simulink subsystem "BatteryHVDetailed_refsub_MultiModule"  (R2022a)
settings: Solver=VariableStepAuto  StartTime=0.0  StopTime=10.0  RelTol=1e-3
undefined symbols (not defined in the file or in its folder): batteryHV_multi_pack1, batteryHV_multi_pack2
libraries: fl_lib x139, nesl_utility x29, batteryModule_lib x12
(part 1 of 3)
settings Model: Creator=jjha  LastModifiedBy=isaacito
settings SolverCC: AlgebraicLoopSolver=TrustRegion
settings DebuggingCC: UnconnectedInputMsg=warning  UnconnectedOutputMsg=warning  UnconnectedLineMsg=warning
settings RTWCC: DLArmComputeVersion=19.05

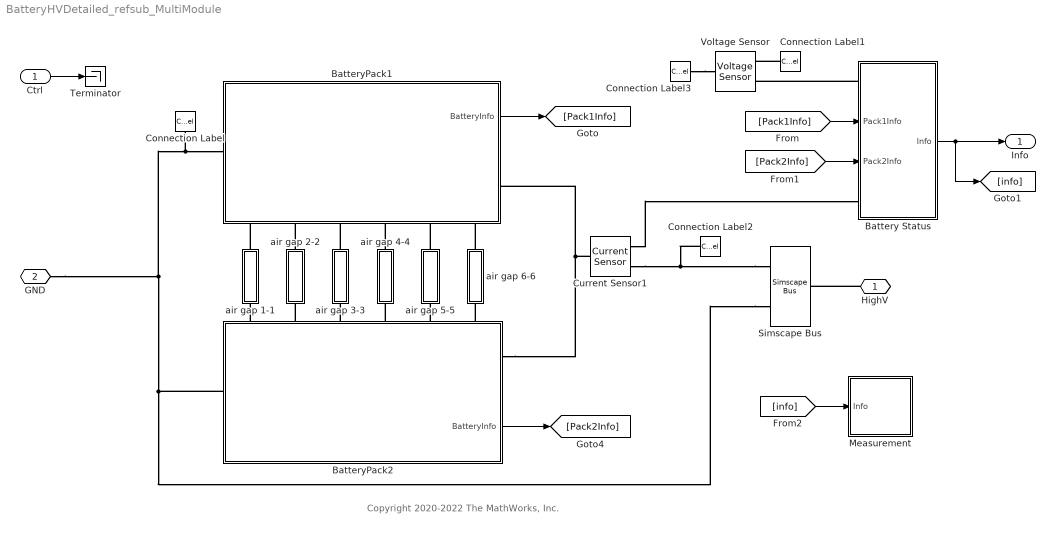
== system BatteryHVDetailed_refsub_MultiModule ==
  note: Copyright 2020-2022 The MathWorks, Inc.
  Ctrl : Inport
  Battery Status : Subsystem
      settings: PortSchema="{\"entries\":[{\"content\":{\"sides\":[{\"content\":{\"connectorIds\":[\"LConn1\",\"In1\",\"In2\",\"LConn2\"]},\"type\":\"ConnectorPlacement.EquallySpacedRectSide\",\"uuid\":\"ed01e2f8-b35f-4cf8-8a1f-a004924ddeb8\"},{\"content\":{\"connectorIds\":[\"Out1\"],\"side\":\"RIGHT\"},\"type\":\"ConnectorPlacement.EquallySpacedRectSide\",\"uuid\":\"7dc9989d-75e9-4ab2-9ee3-28d589c09f12\"},{\"content\":{\"connectorIds\":[],\"side\":\"TOP\"},\"type\":\"ConnectorPlacement.EquallySpacedRectSide\",\"uuid\":\"5d4fb4bf-c728-4f18-a915-de0993398bd4\"},{\"content\":{\"connectorIds\":[],\"side\":\"HIDDEN\"},\"type\":\"ConnectorPlacement.EquallySpacedRectSide\",\"uuid\":\"914bcd26-ac78-4b8d-9b0f-7ad78e1790ea\"}]},\"type\":\"ConnectorPlacement.EquallySpacedConnector\",\"uuid\":\"fc762cf8-918b-4a14-9282-253d1ee4be5d\"}],\"packageUris\":[\"http://schema.mathworks.com/mf0/Connector/R2020b\"],\"version\":\"1.0\"}"
  BatteryPack1 : Subsystem
      settings: PortSchema="{\"entries\":[{\"content\":{\"sides\":[{\"content\":{\"connectorIds\":[\"LConn1\"]},\"type\":\"ConnectorPlacement.EquallySpacedRectSide\",\"uuid\":\"b8d27d12-ba4e-497e-8eeb-93fb9beb614e\"},{\"content\":{\"connectorIds\":[\"Out1\",\"RConn1\"],\"side\":\"RIGHT\"},\"type\":\"ConnectorPlacement.EquallySpacedRectSide\",\"uuid\":\"3a767e09-1002-4db2-833d-9b3c14bcec7d\"},{\"content\":{\"connectorIds\":[],\"side\":\"TOP\"},\"type\":\"ConnectorPlacement.EquallySpacedRectSide\",\"uuid\":\"f8ad4e8a-2322-4ebd-b132-c16be085a9fd\"},{\"content\":{\"connectorIds\":[\"RConn2\",\"RConn3\",\"RConn4\",\"RConn5\",\"RConn6\",\"RConn7\"],\"side\":\"BOTTOM\"},\"type\":\"ConnectorPlacement.EquallySpacedRectSide\",\"uuid\":\"f73fd38f-dbed-4da5-b74f-fbadab7e811a\"},{\"content\":{\"connectorIds\":[],\"side\":\"HIDDEN\"},\"type\":\"ConnectorPlacement.EquallySpacedRectSide\",\"uuid\":\"26d95d03-e87b-489f-a99f-012a8d09d994\"}]},\"type\":\"ConnectorPlacement.EquallySpacedConnector\",\"uuid\":\"7600e896-e4bd-4da6-9432-0a1ab84cea55\"}],\"packageUris\":[\"http://schema.mathworks.com/mf0/Connector/R2020b\"],\"version\":\"1.0\"}"
      mask Display: image('Batterypack_SideView.png'); % Use "Edit Image" on toolstrip to change.
  BatteryPack2 : Subsystem
      settings: PortSchema="{\"entries\":[{\"content\":{\"sides\":[{\"content\":{\"connectorIds\":[\"LConn1\"]},\"type\":\"ConnectorPlacement.EquallySpacedRectSide\",\"uuid\":\"b8d27d12-ba4e-497e-8eeb-93fb9beb614e\"},{\"content\":{\"connectorIds\":[\"RConn1\",\"Out1\"],\"side\":\"RIGHT\"},\"type\":\"ConnectorPlacement.EquallySpacedRectSide\",\"uuid\":\"3a767e09-1002-4db2-833d-9b3c14bcec7d\"},{\"content\":{\"connectorIds\":[\"LConn2\",\"LConn3\",\"LConn4\",\"LConn5\",\"LConn6\",\"LConn7\"],\"side\":\"TOP\"},\"type\":\"ConnectorPlacement.EquallySpacedRectSide\",\"uuid\":\"f8ad4e8a-2322-4ebd-b132-c16be085a9fd\"},{\"content\":{\"connectorIds\":[],\"side\":\"BOTTOM\"},\"type\":\"ConnectorPlacement.EquallySpacedRectSide\",\"uuid\":\"f73fd38f-dbed-4da5-b74f-fbadab7e811a\"},{\"content\":{\"connectorIds\":[],\"side\":\"HIDDEN\"},\"type\":\"ConnectorPlacement.EquallySpacedRectSide\",\"uuid\":\"26d95d03-e87b-489f-a99f-012a8d09d994\"}]},\"type\":\"ConnectorPlacement.EquallySpacedConnector\",\"uuid\":\"7600e896-e4bd-4da6-9432-0a1ab84cea55\"}],\"packageUris\":[\"http://schema.mathworks.com/mf0/Connector/R2020b\"],\"version\":\"1.0\"}"
      mask Display: image('Batterypack_SideView.png'); % Use "Edit Image" on toolstrip to change.
  Connection Label : ConnectionLabel  Label=BatNeg
  Connection Label1 : ConnectionLabel  Label=BatNeg
  Connection Label2 : ConnectionLabel  Label=BatPos
  Connection Label3 : ConnectionLabel  Label=BatPos
  Current Sensor1 : fl_lib/Electrical/Electrical Sensors/Current Sensor
      settings: SourceProductBaseCode=PW,SS,VE
  Measurement : Subsystem
  Simscape Bus : SimscapeBus  HierarchyStrings=plus;minus
  Terminator : Terminator
  Voltage Sensor : fl_lib/Electrical/Electrical Sensors/Voltage Sensor
      settings: SourceProductBaseCode=PW,SS,VE
  air gap 1-1 : Subsystem
  air gap 2-2 : Subsystem
  air gap 3-3 : Subsystem
  air gap 4-4 : Subsystem
  air gap 5-5 : Subsystem
  air gap 6-6 : Subsystem
  HighV : PMIOPort  Side=Right
  GND : PMIOPort  Port=2  Side=Left
  Info : Outport
  wires:
  Battery Status/1(Info) -> Info/1, [info]
  BatteryPack2/1(BatteryInfo) -> [Pack2Info]
  Ctrl/1 -> Terminator/1
  BatteryPack1/1(BatteryInfo) -> [Pack1Info]
  [Pack1Info] -> Battery Status/1(Pack1Info)
  [Pack2Info] -> Battery Status/2(Pack2Info)
  [info] -> Measurement/1(Info)
  connections:
  BatteryPack2/RConn1 -- Current Sensor1/LConn1 -- BatteryPack1/RConn1
  Simscape Bus/LConn2 -- Connection Label/LConn1 -- BatteryPack1/LConn1 -- GND/RConn1 -- BatteryPack2/LConn1
  Simscape Bus/LConn1 -- Connection Label2/LConn1 -- Current Sensor1/RConn2
  HighV/RConn1 -- Simscape Bus/RConn1
  BatteryPack2/LConn7 -- air gap 6-6/RConn1
  Battery Status/LConn1 -- Voltage Sensor/RConn1
  Current Sensor1/RConn1 -- Battery Status/LConn2
  BatteryPack2/LConn2 -- air gap 1-1/RConn1
  BatteryPack2/LConn3 -- air gap 2-2/RConn1
  BatteryPack2/LConn4 -- air gap 3-3/RConn1
  BatteryPack2/LConn5 -- air gap 4-4/RConn1
  BatteryPack2/LConn6 -- air gap 5-5/RConn1
  air gap 5-5/LConn1 -- BatteryPack1/RConn6
  air gap 4-4/LConn1 -- BatteryPack1/RConn5
  air gap 6-6/LConn1 -- BatteryPack1/RConn7
  air gap 2-2/LConn1 -- BatteryPack1/RConn3
  air gap 1-1/LConn1 -- BatteryPack1/RConn2
  air gap 3-3/LConn1 -- BatteryPack1/RConn4
  Connection Label1/LConn1 -- Voltage Sensor/RConn2
  Connection Label3/LConn1 -- Voltage Sensor/LConn1

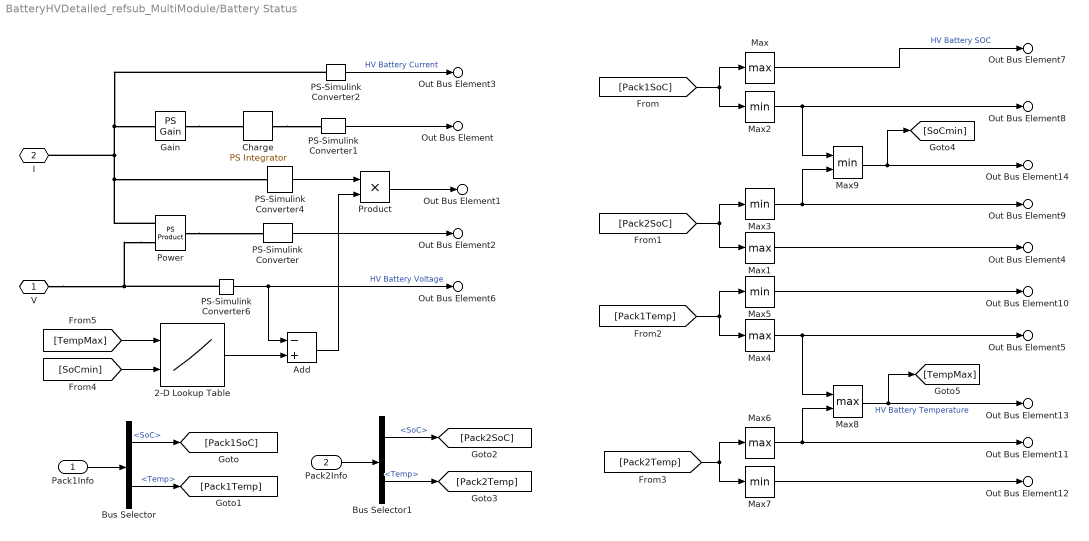
== system BatteryHVDetailed_refsub_MultiModule/Battery Status ==
  Pack1Info : Inport
  Pack2Info : Inport  Port=2
  2-D Lookup Table : Lookup_n-D  BreakpointsForDimension1=batteryHV_multi_pack1.batterySOC_LUT  BreakpointsForDimension2=batteryHV_multi_pack1.batteryTemp_LUT  Table=batteryHV_multi_pack1.batteryEm_LUT  InternalRulePriority=Speed  RndMeth=Simplest
      settings: InputPortMap=u0,u1
  Add : Sum  Inputs=-+
  Bus Selector : BusSelector  OutputSignals=SoC,Temp
  Bus Selector1 : BusSelector  OutputSignals=SoC,Temp
  Charge : fl_lib/Physical Signals/Linear Operators/PS Integrator  reset_method=foundation.enum.IntegratorResetSpec.None  initial_condition_spec=foundation.enum.IntegratorICSpec.Internal  x0=batteryHV_multi_other.batteryPackAhr_ini A*hr
      settings: SourceProductBaseCode=PW,SS,VE
  Gain : fl_lib/Physical Signals/Functions/PS Gain  gain=-1
      settings: AttributesFormatString=%<gain>  SourceProductBaseCode=PW,SS,VE
  Max{,1,4,6} (4 alike) : MinMax  Function=max  ZeroCross=off
  Max{2..3,5,7} (4 alike) : MinMax  ZeroCross=off
  Max8 : MinMax  Function=max  Inputs=2
  Max9 : MinMax  Inputs=2
  PS-Simulink Converter : nesl_utility/PS-Simulink Converter  PhysicalDomain=network_engine_domain  SubClassName=ps_output  LeftPortType=input  RightPortType=output  PseudoPeriodic=off  Frequencies=[]  VectorFormat=1-D array  Unit=kW  AffineConversion=off
      settings: SourceProductBaseCode=SS,PW,VE
  PS-Simulink Converter1 : nesl_utility/PS-Simulink Converter  PhysicalDomain=network_engine_domain  SubClassName=ps_output  LeftPortType=input  RightPortType=output  PseudoPeriodic=off  Frequencies=[]  VectorFormat=1-D array  Unit=A*hr  AffineConversion=off
      settings: SourceProductBaseCode=SS,PW,VE
  PS-Simulink Converter2 : nesl_utility/PS-Simulink Converter  PhysicalDomain=network_engine_domain  SubClassName=ps_output  LeftPortType=input  RightPortType=output  PseudoPeriodic=off  Frequencies=[]  VectorFormat=1-D array  Unit=A  AffineConversion=off
      settings: SourceProductBaseCode=SS,PW,VE
  PS-Simulink Converter4 : nesl_utility/PS-Simulink Converter  PhysicalDomain=network_engine_domain  SubClassName=ps_output  LeftPortType=input  RightPortType=output  PseudoPeriodic=off  Frequencies=[]  VectorFormat=1-D array  Unit=A  AffineConversion=off
      settings: SourceProductBaseCode=SS,PW,VE
  PS-Simulink Converter6 : nesl_utility/PS-Simulink Converter  PhysicalDomain=network_engine_domain  SubClassName=ps_output  LeftPortType=input  RightPortType=output  PseudoPeriodic=off  Frequencies=[]  VectorFormat=1-D array  Unit=V  AffineConversion=off
      settings: SourceProductBaseCode=SS,PW,VE
  Power : fl_lib/Physical Signals/Functions/PS Product
      settings: SourceProductBaseCode=PW,SS,VE
  Product : Product
  V : PMIOPort  Side=Left
  I : PMIOPort  Port=2  Side=Left
  Out Bus Element : Outport  PortName=Info  Element=Charge
      settings: AttributesFormatString=%<Unit>
  Out Bus Element1 : Outport  PortName=Info  Element=PowerLoss
      settings: AttributesFormatString=%<Unit>
  Out Bus Element2 : Outport  PortName=Info  Element=Power
      settings: AttributesFormatString=%<Unit>
  Out Bus Element3 : Outport  PortName=Info  Element=Current
      settings: AttributesFormatString=%<Unit>
  Out Bus Element4 : Outport  PortName=Info  Element=SoC2Max
      settings: AttributesFormatString=%<Unit>
  Out Bus Element5 : Outport  PortName=Info  Element=Temp1Max
      settings: AttributesFormatString=%<Unit>
  Out Bus Element6 : Outport  PortName=Info  Element=Voltage
      settings: AttributesFormatString=%<Unit>
  Out Bus Element7 : Outport  PortName=Info  Element=SoC1Max
      settings: AttributesFormatString=%<Unit>
  Out Bus Element8 : Outport  PortName=Info  Element=SoC1Min
      settings: AttributesFormatString=%<Unit>
  Out Bus Element9 : Outport  PortName=Info  Element=SoC2Min
      settings: AttributesFormatString=%<Unit>
  Out Bus Element10 : Outport  PortName=Info  Element=Temp1Min
      settings: AttributesFormatString=%<Unit>
  Out Bus Element11 : Outport  PortName=Info  Element=Temp2Max
      settings: AttributesFormatString=%<Unit>
  Out Bus Element12 : Outport  PortName=Info  Element=Temp2Min
      settings: AttributesFormatString=%<Unit>
  Out Bus Element13 : Outport  PortName=Info  Element=Temp
      settings: AttributesFormatString=%<Unit>
  Out Bus Element14 : Outport  PortName=Info  Element=SOC
      settings: AttributesFormatString=%<Unit>
  wires:
  Max8/1 -> Out Bus Element13/1, [TempMax]  "HV Battery Temperature"
  Max9/1 -> Out Bus Element14/1, [SoCmin]
  Add/1 -> Product/2
  PS-Simulink Converter4/1 -> Product/1
  2-D Lookup Table/1 -> Add/2
  [TempMax] -> 2-D Lookup Table/1
  [SoCmin] -> 2-D Lookup Table/2
  Max3/1 -> Out Bus Element9/1, Max9/2
  Max6/1 -> Out Bus Element11/1, Max8/2
  Bus Selector1/2 -> [Pack2Temp]  "<Temp>"
  Bus Selector1/1 -> [Pack2SoC]  "<SoC>"
  Bus Selector/2 -> [Pack1Temp]  "<Temp>"
  Bus Selector/1 -> [Pack1SoC]  "<SoC>"
  Pack2Info/1 -> Bus Selector1/1
  Pack1Info/1 -> Bus Selector/1
  PS-Simulink Converter6/1 -> Out Bus Element6/1, Add/1  "HV Battery Voltage"
  PS-Simulink Converter2/1 -> Out Bus Element3/1  "HV Battery Current"
  PS-Simulink Converter/1 -> Out Bus Element2/1
  PS-Simulink Converter1/1 -> Out Bus Element/1
  Product/1 -> Out Bus Element1/1
  [Pack1SoC] -> Max2/1, Max/1
  [Pack2SoC] -> Max1/1, Max3/1
  [Pack1Temp] -> Max4/1, Max5/1
  [Pack2Temp] -> Max7/1, Max6/1
  Max1/1 -> Out Bus Element4/1
  Max/1 -> Out Bus Element7/1  "HV Battery SOC"
  Max2/1 -> Out Bus Element8/1, Max9/1
  Max4/1 -> Out Bus Element5/1, Max8/1
  Max5/1 -> Out Bus Element10/1
  Max7/1 -> Out Bus Element12/1
  connections:
  Gain/RConn1 -- Charge/LConn1
  Charge/RConn1 -- PS-Simulink Converter1/LConn1
  Power/RConn1 -- PS-Simulink Converter/LConn1
  Power/LConn1 -- PS-Simulink Converter6/LConn1 -- V/RConn1
  I/RConn1 -- PS-Simulink Converter4/LConn1 -- Power/LConn2 -- Gain/LConn1 -- PS-Simulink Converter2/LConn1

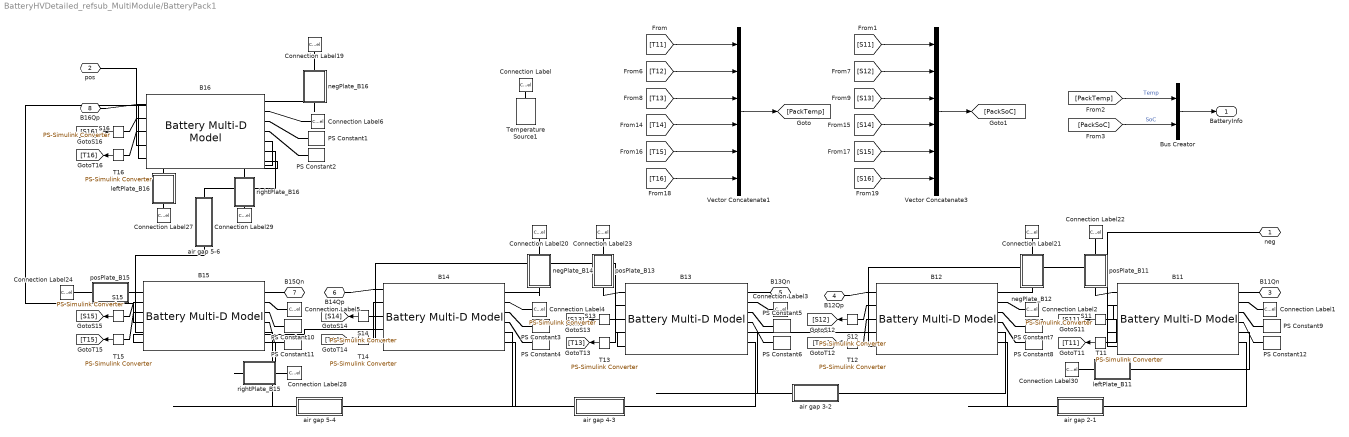
== system BatteryHVDetailed_refsub_MultiModule/BatteryPack1 ==
  B{11..14} (4 alike) : batteryModule_lib/Battery Multi-D Model  modelComplexity=batteryModule.batteryAbstractionLevel.grouped  LUTpointsTemp=batteryHV_multi_pack1.batteryTemp_LUT K  cellAH=batteryHV_multi_pack1.batteryCharge_Ahr A*hr  LUTpointsSOC=batteryHV_multi_pack1.batterySOC_LUT  V0_mat=batteryHV_multi_pack1.batteryEm_LUT V  prm_dir=ee.enum.battery.prm_dir.noCurrentDirectionality  R0_mat=batteryHV_multi_pack1.batteryR0_LUT Ohm  R0_dis_mat=[.03, .015, .002; .04, .017, .008; .039, .012, .006; .027, .013, .021] Ohm  R0_ch_mat=[.03, .015, .002; .04, .017, .008; .039, .012, .006; .027, .013, .021] Ohm  prm_leak=ee.enum.battery.prm_leak.disabled  Rleak_vec=[8000, 7000, 6000] Ohm  extrapolation_option=simscape.enum.extrapolation.nearest  prm_dyn=ee.enum.battery.prm_dyn.rc1  R1_mat=batteryHV_multi_pack1.batteryR1_LUT Ohm  tau1_mat=batteryHV_multi_pack1.batteryTau1_LUT s  R2_mat=[.014, .382, .407; .028, .006, .007; .014, .007, .006; .333, .956, .912] Ohm  tau2_mat=[1, 44, 5644; 11, 24, 506; 2, 14, 330; 3310, 13419, 30216] s  R3_mat=[.014, .382, .407; .028, .006, .007; .014, .007, .006; .333, .956, .912] Ohm  tau3_mat=[1, 44, 5644; 11, 24, 506; 2, 14, 330; 3310, 13419, 30216] s  R4_mat=[.014, .382, .407; .028, .006, .007; .014, .007, .006; .333, .956, .912] Ohm  tau4_mat=[1, 44, 5644; 11, 24, 506; 2, 14, 330; 3310, 13419, 30216] s  R5_mat=[.014, .382, .407; .028, .006, .007; .014, .007, .006; .333, .956, .912] Ohm  tau5_mat=[1, 44, 5644; 11, 24, 506; 2, 14, 330; 3310, 13419, 30216] s  prm_fade=ee.enum.battery.prm_fade.equations  N0=100  dV0=0  dR0=0  dAH=0  dRleak=0  dR1=0  dR2=0  dR3=0  dR4=0  dR5=0  N0vec=[100, 200, 300]  Tfadevec=[298.15, 323.15] K  dV0vec=[0, 0, 0]  dR0vec=[0, 0, 0]  dAHvec=[0, 0, 0]  dRleakvec=[0, 0, 0]  dR1vec=[0, 0, 0]  dR2vec=[0, 0, 0]  dR3vec=[0, 0, 0]  dR4vec=[0, 0, 0]  dR5vec=[0, 0, 0]  dV0mat=[0, 0; 0, 0; 0, 0]  dR0mat=[0, 0; 0, 0; 0, 0]  dAHmat=[0, 0; 0, 0; 0, 0]  dRleakmat=[0, 0; 0, 0; 0, 0]  dR1mat=[0, 0; 0, 0; 0, 0]  dR2mat=[0, 0; 0, 0; 0, 0]  dR3mat=[0, 0; 0, 0; 0, 0]  dR4mat=[0, 0; 0, 0; 0, 0]  dR5mat=[0, 0; 0, 0; 0, 0]  cellThermalMass=batteryHV_multi_pack1.batteryCell_mass*batteryHV_multi_pack1.batteryCell_cp J/K  cellThermalCond=batteryHV_multi_pack1.batteryThermal_K1 W/(m*K)  cellThermalCond_inPlane=batteryHV_multi_pack1.batteryThermal_K2 W/(m*K)  Ns=batteryHV_multi_pack1.batteryNs  Np=batteryHV_multi_pack1.batteryNp  cellTypeSelection=batteryModule.batteryTypeSelection.pouch  cellHeight=batteryHV_multi_pack1.batteryCell_H m  cellWidth=batteryHV_multi_pack1.batteryCell_W m  cellThickness=batteryHV_multi_pack1.batteryCell_T m  cellDiameter=0.018 m  cellCylinLine=3  moduleExternalR=batteryHV_multi_pack1.battery_extR Ohm  moduleCellBalancing=batteryModule.batteryCellBalancing.none  passiveShuntR=50 Ohm  passiveSWclosedR=0.01 Ohm  passiveSWopenCond=1e-8 1/Ohm  passiveSWthreshold=0.5  moduleCellVoltages=batteryModule.batteryCellVoltages.no  thermalManagement=batteryModule.batteryCoolingSystem.thermalPort  cellHeatTrCoeff=1 W/(m^2 * K)  thermal_moduleBottom=batteryModule.batteryThermalPortSelection.thermalLUT  htc_bottom=1 W/(m^2 * K)  moduleCooling_b=batteryHV_multi_pack1.batteryModuleBottomHTC W/K  LUTpointsFlowrate_b=batteryHV_multi_pack1.batteryCoolant_flow kg/s  LUTpointsTemp_b=batteryHV_multi_pack1.batteryTemp_LUT K  thermal_moduleTop=batteryModule.batteryThermalPortSelection.convectionBC  htc_top=batteryHV_multi_pack1.batteryModuleTopHTC W/(m^2 * K)  moduleCooling_t=batteryHV_multi_pack1.batteryCoolantHTC W/K  LUTpointsFlowrate_t=batteryHV_multi_pack1.batteryCoolant_flow kg/s  LUTpointsTemp_t=batteryHV_multi_pack1.batteryTemp_LUT K  thermal_moduleRight=batteryModule.batteryThermalPortSelection.thermalPortLumped  htc_right=1 W/(m^2 * K)  moduleCooling_r=zeros(3,6,batteryHV_multi_pack1.batteryNs*batteryHV_multi_pack1.batteryNp) W/K  LUTpointsFlowrate_r=[.01, .02, .03, .04, .05, .06] kg/s  LUTpointsTemp_r=[273.15, 298.15, 323.15] K  thermal_moduleLeft=batteryModule.batteryThermalPortSelection.thermalPortLumped  htc_left=1 W/(m^2 * K)  moduleCooling_l=zeros(3,6,batteryHV_multi_pack1.batteryNs*batteryHV_multi_pack1.batteryNp) W/K  LUTpointsFlowrate_l=[.01, .02, .03, .04, .05, .06] kg/s  LUTpointsTemp_l=[273.15, 298.15, 323.15] K  thermal_modulePos=batteryModule.batteryThermalPortSelection.thermalPortLumped  htc_pos=1 W/(m^2 * K)  moduleCooling_p=zeros(3,6,batteryHV_multi_pack1.batteryNs*batteryHV_multi_pack1.batteryNp) W/K  LUTpointsFlowrate_p=[.01, .02, .03, .04, .05, .06] kg/s  LUTpointsTemp_p=[273.15, 298.15, 323.15] K  thermal_moduleNeg=batteryModule.batteryThermalPortSelection.thermalPortLumped  htc_neg=1 W/(m^2 * K)  moduleCooling_n=zeros(3,6,batteryHV_multi_pack1.batteryNs*batteryHV_multi_pack1.batteryNp) W/K  LUTpointsFlowrate_n=[.01, .02, .03, .04, .05, .06] kg/s  LUTpointsTemp_n=[273.15, 298.15, 323.15] K  moduleExtHeat=batteryHV_multi_pack1.batteryModuleExtHeat W  cellTemp=batteryHV_multi_pack1.batteryModuleCellT_ini K  cellSOC=batteryHV_multi_pack1.batteryModuleCellSOC_ini  moduleCellAHpercentVar=batteryHV_multi_pack1.batteryModuleCellAhr_ini  moduleCellLeakPercentVar=ones(1, 10)  moduleCellR0PercentVar=batteryHV_multi_pack1.batteryModuleCellR0_ini
      settings: InternalSimscapePortConfiguration="{\"Bottom\":[{\"id\":\"Ql\",\"label\":\"Ql\",\"type\":\"foundation.thermal.thermal\"},{\"id\":\"Qr\",\"label\":\"Qr\",\"type\":\"foundation.thermal.thermal\"}],\"Left\":[{\"id\":\"Qp\",\"label\":\"Qp\",\"type\":\"foundation.thermal.thermal\"},{\"id\":\"outputCellSOC\",\"label\":\"SOC\",\"type\":\"output\"},{\"id\":\"outputCellTemp\",\"label\":\"Temp\",\"type\":\"output\"}],\"Right\":[{\"id\":\"Qn\",\"label\":\"Qn\",\"type\":\"foundation.thermal.thermal\"},{\"id\":\"H\",\"label\":\"Amb\",\"type\":\"foundation.thermal.thermal\"},{\"id\":\"frac_b\",\"label\":\"FlwR\",\"type\":\"input\"},{\"id\":\"delT_b\",\"label\":\"FlwT\",\"type\":\"input\"}],\"Top\":[{\"id\":\"p\",\"label\":\"pos\",\"type\":\"foundation.electrical.electrical\"},{\"id\":\"n\",\"label\":\"neg\",\"type\":\"foundation.electrical.electrical\"}]}"
  B15 : batteryModule_lib/Battery Multi-D Model  modelComplexity=batteryModule.batteryAbstractionLevel.grouped  LUTpointsTemp=batteryHV_multi_pack1.batteryTemp_LUT K  cellAH=batteryHV_multi_pack1.batteryCharge_Ahr A*hr  LUTpointsSOC=batteryHV_multi_pack1.batterySOC_LUT  V0_mat=batteryHV_multi_pack1.batteryEm_LUT V  prm_dir=ee.enum.battery.prm_dir.noCurrentDirectionality  R0_mat=batteryHV_multi_pack1.batteryR0_LUT Ohm  R0_dis_mat=[.03, .015, .002; .04, .017, .008; .039, .012, .006; .027, .013, .021] Ohm  R0_ch_mat=[.03, .015, .002; .04, .017, .008; .039, .012, .006; .027, .013, .021] Ohm  prm_leak=ee.enum.battery.prm_leak.disabled  Rleak_vec=[8000, 7000, 6000] Ohm  extrapolation_option=simscape.enum.extrapolation.nearest  prm_dyn=ee.enum.battery.prm_dyn.rc1  R1_mat=batteryHV_multi_pack1.batteryR1_LUT Ohm  tau1_mat=batteryHV_multi_pack1.batteryTau1_LUT s  R2_mat=[.014, .382, .407; .028, .006, .007; .014, .007, .006; .333, .956, .912] Ohm  tau2_mat=[1, 44, 5644; 11, 24, 506; 2, 14, 330; 3310, 13419, 30216] s  R3_mat=[.014, .382, .407; .028, .006, .007; .014, .007, .006; .333, .956, .912] Ohm  tau3_mat=[1, 44, 5644; 11, 24, 506; 2, 14, 330; 3310, 13419, 30216] s  R4_mat=[.014, .382, .407; .028, .006, .007; .014, .007, .006; .333, .956, .912] Ohm  tau4_mat=[1, 44, 5644; 11, 24, 506; 2, 14, 330; 3310, 13419, 30216] s  R5_mat=[.014, .382, .407; .028, .006, .007; .014, .007, .006; .333, .956, .912] Ohm  tau5_mat=[1, 44, 5644; 11, 24, 506; 2, 14, 330; 3310, 13419, 30216] s  prm_fade=ee.enum.battery.prm_fade.equations  N0=100  dV0=0  dR0=0  dAH=0  dRleak=0  dR1=0  dR2=0  dR3=0  dR4=0  dR5=0  N0vec=[100, 200, 300]  Tfadevec=[298.15, 323.15] K  dV0vec=[0, 0, 0]  dR0vec=[0, 0, 0]  dAHvec=[0, 0, 0]  dRleakvec=[0, 0, 0]  dR1vec=[0, 0, 0]  dR2vec=[0, 0, 0]  dR3vec=[0, 0, 0]  dR4vec=[0, 0, 0]  dR5vec=[0, 0, 0]  dV0mat=[0, 0; 0, 0; 0, 0]  dR0mat=[0, 0; 0, 0; 0, 0]  dAHmat=[0, 0; 0, 0; 0, 0]  dRleakmat=[0, 0; 0, 0; 0, 0]  dR1mat=[0, 0; 0, 0; 0, 0]  dR2mat=[0, 0; 0, 0; 0, 0]  dR3mat=[0, 0; 0, 0; 0, 0]  dR4mat=[0, 0; 0, 0; 0, 0]  dR5mat=[0, 0; 0, 0; 0, 0]  cellThermalMass=batteryHV_multi_pack1.batteryCell_mass*batteryHV_multi_pack1.batteryCell_cp J/K  cellThermalCond=batteryHV_multi_pack1.batteryThermal_K1 W/(m*K)  cellThermalCond_inPlane=batteryHV_multi_pack1.batteryThermal_K2 W/(m*K)  Ns=batteryHV_multi_pack1.batteryNs  Np=batteryHV_multi_pack1.batteryNp  cellTypeSelection=batteryModule.batteryTypeSelection.pouch  cellHeight=batteryHV_multi_pack1.batteryCell_H m  cellWidth=batteryHV_multi_pack1.batteryCell_W m  cellThickness=batteryHV_multi_pack1.batteryCell_T m  cellDiameter=0.018 m  cellCylinLine=3  moduleExternalR=batteryHV_multi_pack1.battery_extR Ohm  moduleCellBalancing=batteryModule.batteryCellBalancing.none  passiveShuntR=50 Ohm  passiveSWclosedR=0.01 Ohm  passiveSWopenCond=1e-8 1/Ohm  passiveSWthreshold=0.5  moduleCellVoltages=batteryModule.batteryCellVoltages.no  thermalManagement=batteryModule.batteryCoolingSystem.thermalPort  cellHeatTrCoeff=1 W/(m^2 * K)  thermal_moduleBottom=batteryModule.batteryThermalPortSelection.thermalLUT  htc_bottom=1 W/(m^2 * K)  moduleCooling_b=batteryHV_multi_pack1.batteryModuleBottomHTC W/K  LUTpointsFlowrate_b=batteryHV_multi_pack1.batteryCoolant_flow kg/s  LUTpointsTemp_b=batteryHV_multi_pack1.batteryTemp_LUT K  thermal_moduleTop=batteryModule.batteryThermalPortSelection.thermalPortLumped  htc_top=batteryHV_multi_pack1.batteryModuleTopHTC W/(m^2 * K)  moduleCooling_t=batteryHV_multi_pack1.batteryCoolantHTC W/K  LUTpointsFlowrate_t=batteryHV_multi_pack1.batteryCoolant_flow kg/s  LUTpointsTemp_t=batteryHV_multi_pack1.batteryTemp_LUT K  thermal_moduleRight=batteryModule.batteryThermalPortSelection.thermalPortLumped  htc_right=1 W/(m^2 * K)  moduleCooling_r=zeros(3,6,batteryHV_multi_pack1.batteryNs*batteryHV_multi_pack1.batteryNp) W/K  LUTpointsFlowrate_r=[.01, .02, .03, .04, .05, .06] kg/s  LUTpointsTemp_r=[273.15, 298.15, 323.15] K  thermal_moduleLeft=batteryModule.batteryThermalPortSelection.thermalPortLumped  htc_left=1 W/(m^2 * K)  moduleCooling_l=zeros(3,6,batteryHV_multi_pack1.batteryNs*batteryHV_multi_pack1.batteryNp) W/K  LUTpointsFlowrate_l=[.01, .02, .03, .04, .05, .06] kg/s  LUTpointsTemp_l=[273.15, 298.15, 323.15] K  thermal_modulePos=batteryModule.batteryThermalPortSelection.thermalPortLumped  htc_pos=1 W/(m^2 * K)  moduleCooling_p=zeros(3,6,batteryHV_multi_pack1.batteryNs*batteryHV_multi_pack1.batteryNp) W/K  LUTpointsFlowrate_p=[.01, .02, .03, .04, .05, .06] kg/s  LUTpointsTemp_p=[273.15, 298.15, 323.15] K  thermal_moduleNeg=batteryModule.batteryThermalPortSelection.thermalPortLumped  htc_neg=1 W/(m^2 * K)  moduleCooling_n=zeros(3,6,batteryHV_multi_pack1.batteryNs*batteryHV_multi_pack1.batteryNp) W/K  LUTpointsFlowrate_n=[.01, .02, .03, .04, .05, .06] kg/s  LUTpointsTemp_n=[273.15, 298.15, 323.15] K  moduleExtHeat=batteryHV_multi_pack1.batteryModuleExtHeat W  cellTemp=batteryHV_multi_pack1.batteryModuleCellT_ini K  cellSOC=batteryHV_multi_pack1.batteryModuleCellSOC_ini  moduleCellAHpercentVar=batteryHV_multi_pack1.batteryModuleCellAhr_ini  moduleCellLeakPercentVar=ones(1, 10)  moduleCellR0PercentVar=batteryHV_multi_pack1.batteryModuleCellR0_ini
      settings: InternalSimscapePortConfiguration="{\"Bottom\":[{\"id\":\"Ql\",\"label\":\"Ql\",\"type\":\"foundation.thermal.thermal\"},{\"id\":\"Qr\",\"label\":\"Qr\",\"type\":\"foundation.thermal.thermal\"}],\"Left\":[{\"id\":\"Qp\",\"label\":\"Qp\",\"type\":\"foundation.thermal.thermal\"},{\"id\":\"outputCellSOC\",\"label\":\"SOC\",\"type\":\"output\"},{\"id\":\"outputCellTemp\",\"label\":\"Temp\",\"type\":\"output\"}],\"Right\":[{\"id\":\"Qn\",\"label\":\"Qn\",\"type\":\"foundation.thermal.thermal\"},{\"id\":\"H\",\"label\":\"Amb\",\"type\":\"foundation.thermal.thermal\"},{\"id\":\"frac_b\",\"label\":\"FlwR\",\"type\":\"input\"},{\"id\":\"delT_b\",\"label\":\"FlwT\",\"type\":\"input\"}],\"Top\":[{\"id\":\"p\",\"label\":\"pos\",\"type\":\"foundation.electrical.electrical\"},{\"id\":\"Qt\",\"label\":\"Qt\",\"type\":\"foundation.thermal.thermal\"},{\"id\":\"n\",\"label\":\"neg\",\"type\":\"foundation.electrical.electrical\"}]}"
  B16 : batteryModule_lib/Battery Multi-D Model  modelComplexity=batteryModule.batteryAbstractionLevel.grouped  LUTpointsTemp=batteryHV_multi_pack1.batteryTemp_LUT K  cellAH=batteryHV_multi_pack1.batteryCharge_Ahr A*hr  LUTpointsSOC=batteryHV_multi_pack1.batterySOC_LUT  V0_mat=batteryHV_multi_pack1.batteryEm_LUT V  prm_dir=ee.enum.battery.prm_dir.noCurrentDirectionality  R0_mat=batteryHV_multi_pack1.batteryR0_LUT Ohm  R0_dis_mat=[.03, .015, .002; .04, .017, .008; .039, .012, .006; .027, .013, .021] Ohm  R0_ch_mat=[.03, .015, .002; .04, .017, .008; .039, .012, .006; .027, .013, .021] Ohm  prm_leak=ee.enum.battery.prm_leak.disabled  Rleak_vec=[8000, 7000, 6000] Ohm  extrapolation_option=simscape.enum.extrapolation.nearest  prm_dyn=ee.enum.battery.prm_dyn.rc1  R1_mat=batteryHV_multi_pack1.batteryR1_LUT Ohm  tau1_mat=batteryHV_multi_pack1.batteryTau1_LUT s  R2_mat=[.014, .382, .407; .028, .006, .007; .014, .007, .006; .333, .956, .912] Ohm  tau2_mat=[1, 44, 5644; 11, 24, 506; 2, 14, 330; 3310, 13419, 30216] s  R3_mat=[.014, .382, .407; .028, .006, .007; .014, .007, .006; .333, .956, .912] Ohm  tau3_mat=[1, 44, 5644; 11, 24, 506; 2, 14, 330; 3310, 13419, 30216] s  R4_mat=[.014, .382, .407; .028, .006, .007; .014, .007, .006; .333, .956, .912] Ohm  tau4_mat=[1, 44, 5644; 11, 24, 506; 2, 14, 330; 3310, 13419, 30216] s  R5_mat=[.014, .382, .407; .028, .006, .007; .014, .007, .006; .333, .956, .912] Ohm  tau5_mat=[1, 44, 5644; 11, 24, 506; 2, 14, 330; 3310, 13419, 30216] s  prm_fade=ee.enum.battery.prm_fade.equations  N0=100  dV0=0  dR0=0  dAH=0  dRleak=0  dR1=0  dR2=0  dR3=0  dR4=0  dR5=0  N0vec=[100, 200, 300]  Tfadevec=[298.15, 323.15] K  dV0vec=[0, 0, 0]  dR0vec=[0, 0, 0]  dAHvec=[0, 0, 0]  dRleakvec=[0, 0, 0]  dR1vec=[0, 0, 0]  dR2vec=[0, 0, 0]  dR3vec=[0, 0, 0]  dR4vec=[0, 0, 0]  dR5vec=[0, 0, 0]  dV0mat=[0, 0; 0, 0; 0, 0]  dR0mat=[0, 0; 0, 0; 0, 0]  dAHmat=[0, 0; 0, 0; 0, 0]  dRleakmat=[0, 0; 0, 0; 0, 0]  dR1mat=[0, 0; 0, 0; 0, 0]  dR2mat=[0, 0; 0, 0; 0, 0]  dR3mat=[0, 0; 0, 0; 0, 0]  dR4mat=[0, 0; 0, 0; 0, 0]  dR5mat=[0, 0; 0, 0; 0, 0]  cellThermalMass=batteryHV_multi_pack1.batteryCell_mass*batteryHV_multi_pack1.batteryCell_cp J/K  cellThermalCond=batteryHV_multi_pack1.batteryThermal_K1 W/(m*K)  cellThermalCond_inPlane=batteryHV_multi_pack1.batteryThermal_K2 W/(m*K)  Ns=batteryHV_multi_pack1.batteryNs  Np=batteryHV_multi_pack1.batteryNp  cellTypeSelection=batteryModule.batteryTypeSelection.pouch  cellHeight=batteryHV_multi_pack1.batteryCell_H m  cellWidth=batteryHV_multi_pack1.batteryCell_W m  cellThickness=batteryHV_multi_pack1.batteryCell_T m  cellDiameter=0.018 m  cellCylinLine=3  moduleExternalR=batteryHV_multi_pack1.battery_extR Ohm  moduleCellBalancing=batteryModule.batteryCellBalancing.none  passiveShuntR=50 Ohm  passiveSWclosedR=0.01 Ohm  passiveSWopenCond=1e-8 1/Ohm  passiveSWthreshold=0.5  moduleCellVoltages=batteryModule.batteryCellVoltages.no  thermalManagement=batteryModule.batteryCoolingSystem.thermalPort  cellHeatTrCoeff=1 W/(m^2 * K)  thermal_moduleBottom=batteryModule.batteryThermalPortSelection.thermalPortLumped  htc_bottom=1 W/(m^2 * K)  moduleCooling_b=batteryHV_multi_pack1.batteryModuleBottomHTC W/K  LUTpointsFlowrate_b=batteryHV_multi_pack1.batteryCoolant_flow kg/s  LUTpointsTemp_b=batteryHV_multi_pack1.batteryTemp_LUT K  thermal_moduleTop=batteryModule.batteryThermalPortSelection.thermalLUT  htc_top=batteryHV_multi_pack1.batteryModuleTopHTC W/(m^2 * K)  moduleCooling_t=batteryHV_multi_pack1.batteryCoolantHTC W/K  LUTpointsFlowrate_t=batteryHV_multi_pack1.batteryCoolant_flow kg/s  LUTpointsTemp_t=batteryHV_multi_pack1.batteryTemp_LUT K  thermal_moduleRight=batteryModule.batteryThermalPortSelection.thermalPortLumped  htc_right=1 W/(m^2 * K)  moduleCooling_r=zeros(3,6,batteryHV_multi_pack1.batteryNs*batteryHV_multi_pack1.batteryNp) W/K  LUTpointsFlowrate_r=[.01, .02, .03, .04, .05, .06] kg/s  LUTpointsTemp_r=[273.15, 298.15, 323.15] K  thermal_moduleLeft=batteryModule.batteryThermalPortSelection.thermalPortLumped  htc_left=1 W/(m^2 * K)  moduleCooling_l=zeros(3,6,batteryHV_multi_pack1.batteryNs*batteryHV_multi_pack1.batteryNp) W/K  LUTpointsFlowrate_l=[.01, .02, .03, .04, .05, .06] kg/s  LUTpointsTemp_l=[273.15, 298.15, 323.15] K  thermal_modulePos=batteryModule.batteryThermalPortSelection.thermalPortLumped  htc_pos=1 W/(m^2 * K)  moduleCooling_p=zeros(3,6,batteryHV_multi_pack1.batteryNs*batteryHV_multi_pack1.batteryNp) W/K  LUTpointsFlowrate_p=[.01, .02, .03, .04, .05, .06] kg/s  LUTpointsTemp_p=[273.15, 298.15, 323.15] K  thermal_moduleNeg=batteryModule.batteryThermalPortSelection.thermalPortLumped  htc_neg=1 W/(m^2 * K)  moduleCooling_n=zeros(3,6,batteryHV_multi_pack1.batteryNs*batteryHV_multi_pack1.batteryNp) W/K  LUTpointsFlowrate_n=[.01, .02, .03, .04, .05, .06] kg/s  LUTpointsTemp_n=[273.15, 298.15, 323.15] K  moduleExtHeat=batteryHV_multi_pack1.batteryModuleExtHeat W  cellTemp=batteryHV_multi_pack1.batteryModuleCellT_ini K  cellSOC=batteryHV_multi_pack1.batteryModuleCellSOC_ini  moduleCellAHpercentVar=batteryHV_multi_pack1.batteryModuleCellAhr_ini  moduleCellLeakPercentVar=ones(1, 10)  moduleCellR0PercentVar=batteryHV_multi_pack1.batteryModuleCellR0_ini
      settings: InternalSimscapePortConfiguration="{\"Bottom\":[{\"id\":\"Ql\",\"label\":\"Ql\",\"type\":\"foundation.thermal.thermal\"},{\"id\":\"Qb\",\"label\":\"Qb\",\"type\":\"foundation.thermal.thermal\"},{\"id\":\"Qr\",\"label\":\"Qr\",\"type\":\"foundation.thermal.thermal\"}],\"Left\":[{\"id\":\"Qp\",\"label\":\"Qp\",\"type\":\"foundation.thermal.thermal\"},{\"id\":\"outputCellSOC\",\"label\":\"SOC\",\"type\":\"output\"},{\"id\":\"outputCellTemp\",\"label\":\"Temp\",\"type\":\"output\"}],\"Right\":[{\"id\":\"Qn\",\"label\":\"Qn\",\"type\":\"foundation.thermal.thermal\"},{\"id\":\"H\",\"label\":\"Amb\",\"type\":\"foundation.thermal.thermal\"},{\"id\":\"frac_t\",\"label\":\"FlwR\",\"type\":\"input\"},{\"id\":\"delT_t\",\"label\":\"FlwT\",\"type\":\"input\"}],\"Top\":[{\"id\":\"p\",\"label\":\"pos\",\"type\":\"foundation.electrical.electrical\"},{\"id\":\"n\",\"label\":\"neg\",\"type\":\"foundation.electrical.electrical\"}]}"
  Bus Creator : BusCreator  Inputs=2
  Connection Label{,1..6,19..24,27..30} (17 alike) : ConnectionLabel  Label=Amb
  PS Constant{1,3,5,7,9..10} (6 alike) : fl_lib/Physical Signals/Sources/PS Constant  constant=batteryHV_multi_other.batteryCoolantFlwR
      settings: SourceProductBaseCode=PW,SS,VE
  PS Constant{2,4,6,8,11..12} (6 alike) : fl_lib/Physical Signals/Sources/PS Constant  constant=batteryHV_multi_other.batteryCoolantFlwT K
      settings: SourceProductBaseCode=PW,SS,VE
  S{11..16} (6 alike) : nesl_utility/PS-Simulink Converter  PhysicalDomain=network_engine_domain  SubClassName=ps_output  LeftPortType=input  RightPortType=output  PseudoPeriodic=off  Frequencies=[]  VectorFormat=1-D array  Unit=1  AffineConversion=off
      settings: SourceProductBaseCode=SS,PW,VE
  T{11..16} (6 alike) : nesl_utility/PS-Simulink Converter  PhysicalDomain=network_engine_domain  SubClassName=ps_output  LeftPortType=input  RightPortType=output  PseudoPeriodic=off  Frequencies=[]  VectorFormat=1-D array  Unit=K  AffineConversion=off
      settings: SourceProductBaseCode=SS,PW,VE
  Temperature Source1 : fl_lib/Thermal/Thermal Sources/Temperature Source  temperature=batteryHV_multi_other.AmbTemp_K K
      settings: SourceProductBaseCode=PW,SS,VE
  Vector Concatenate1 : Concatenate  NumInputs=6
  Vector Concatenate3 : Concatenate  NumInputs=6
  air gap 2-1 : Subsystem
  air gap 3-2 : Subsystem
  air gap 4-3 : Subsystem
  air gap 5-4 : Subsystem
  air gap 5-6 : Subsystem
  leftPlate_B11 : Subsystem
  leftPlate_B16 : Subsystem
  negPlate_B12 : Subsystem
  negPlate_B14 : Subsystem
  negPlate_B16 : Subsystem
  posPlate_B11 : Subsystem
  posPlate_B13 : Subsystem
  posPlate_B15 : Subsystem
  rightPlate_B15 : Subsystem
  rightPlate_B16 : Subsystem
  neg : PMIOPort  Side=Left
  pos : PMIOPort  Port=2  Side=Right
  B11Qn : PMIOPort  Port=3  Side=Right
  B12Qp : PMIOPort  Port=4  Side=Right
  B13Qn : PMIOPort  Port=5  Side=Right
  B14Qp : PMIOPort  Port=6  Side=Right
  B15Qn : PMIOPort  Port=7  Side=Right
  B16Qp : PMIOPort  Port=8  Side=Right
  BatteryInfo : Outport
  wires:
  [PackSoC] -> Bus Creator/2  "SoC"
  [PackTemp] -> Bus Creator/1  "Temp"
  Bus Creator/1 -> BatteryInfo/1
  T16/1 -> [T16]
  S11/1 -> [S11]
  S13/1 -> [S13]
  S12/1 -> [S12]
  T12/1 -> [T12]
  T11/1 -> [T11]
  T14/1 -> [T14]
  T13/1 -> [T13]
  S14/1 -> [S14]
  S15/1 -> [S15]
  T15/1 -> [T15]
  [S16] -> Vector Concatenate3/6
  [S15] -> Vector Concatenate3/5
  [S11] -> Vector Concatenate3/1
  Vector Concatenate1/1 -> [PackTemp]
  Vector Concatenate3/1 -> [PackSoC]
  [S14] -> Vector Concatenate3/4
  [T14] -> Vector Concatenate1/4
  [T11] -> Vector Concatenate1/1
  [T15] -> Vector Concatenate1/5
  [T13] -> Vector Concatenate1/3
  [T12] -> Vector Concatenate1/2
  [S13] -> Vector Concatenate3/3
  [T16] -> Vector Concatenate1/6
  [S12] -> Vector Concatenate3/2
  S16/1 -> [S16]
  connections:
  air gap 2-1/RConn1 -- B11/RConn6
  air gap 3-2/RConn1 -- B12/RConn5
  air gap 4-3/RConn1 -- B13/RConn6
  air gap 5-4/RConn1 -- B14/RConn5
  leftPlate_B11/RConn1 -- B11/RConn5
  Connection Label30/LConn1 -- leftPlate_B11/LConn1
  negPlate_B12/LConn1 -- Connection Label21/LConn1
  B12/RConn1 -- negPlate_B12/RConn1
  negPlate_B14/LConn1 -- Connection Label20/LConn1
  negPlate_B14/RConn1 -- B14/RConn1
  leftPlate_B16/RConn1 -- B16/RConn5
  Connection Label27/LConn1 -- leftPlate_B16/LConn1
  negPlate_B16/LConn1 -- Connection Label19/LConn1
  negPlate_B16/RConn1 -- B16/RConn1
  B16/LConn3 -- T16/LConn1
  B14/LConn2 -- S14/LConn1
  Connection Label5/LConn1 -- B15/RConn2
  air gap 5-4/LConn1 -- B15/RConn5
  B13/LConn4 -- B14/LConn5
  air gap 5-6/LConn1 -- B15/LConn5
  Connection Label4/LConn1 -- B14/RConn2
  B15/LConn2 -- S15/LConn1
  posPlate_B15/RConn1 -- B15/LConn1
  B15/LConn3 -- T15/LConn1
  B15/LConn6 -- B14/LConn4
  Connection Label24/LConn1 -- posPlate_B15/LConn1
  posPlate_B11/RConn1 -- B11/LConn1
  air gap 5-6/RConn1 -- B16/RConn6
  B11/RConn2 -- Connection Label1/LConn1
  B13/LConn3 -- T13/LConn1
  posPlate_B13/LConn1 -- Connection Label23/LConn1
  B13/RConn2 -- Connection Label3/LConn1
  rightPlate_B15/LConn1 -- Connection Label28/LConn1
  air gap 2-1/LConn1 -- B12/RConn6
  B15/LConn4 -- B16/LConn5
  rightPlate_B15/RConn1 -- B15/RConn6
  Connection Label29/LConn1 -- rightPlate_B16/LConn1
  B11/LConn2 -- S11/LConn1
  B15/RConn1 -- B15Qn/RConn1
  rightPlate_B16/RConn1 -- B16/RConn7
  posPlate_B13/RConn1 -- B13/LConn1
  Connection Label6/LConn1 -- B16/RConn2
  B12/LConn3 -- T12/LConn1
  B11/LConn4 -- B12/LConn5
  B11/LConn3 -- T11/LConn1
  B12/RConn2 -- Connection Label2/LConn1
  air gap 4-3/LConn1 -- B14/RConn6
  B12/LConn2 -- S12/LConn1
  B13/LConn2 -- S13/LConn1
  B14/LConn3 -- T14/LConn1
  B12/LConn4 -- B13/LConn5
  air gap 3-2/LConn1 -- B13/RConn5
  posPlate_B11/LConn1 -- Connection Label22/LConn1
  B16/LConn1 -- B16Qp/RConn1
  B11/LConn5 -- neg/RConn1
  B16/LConn2 -- S16/LConn1
  B11/RConn1 -- B11Qn/RConn1
  B13/RConn1 -- B13Qn/RConn1
  B14/LConn1 -- B14Qp/RConn1
  B16/LConn4 -- pos/RConn1
  B12/LConn1 -- B12Qp/RConn1
  Connection Label/LConn1 -- Temperature Source1/LConn1
  PS Constant1/RConn1 -- B16/RConn3
  PS Constant2/RConn1 -- B16/RConn4
  PS Constant10/RConn1 -- B15/RConn3
  PS Constant11/RConn1 -- B15/RConn4
  PS Constant3/RConn1 -- B14/RConn3
  PS Constant4/RConn1 -- B14/RConn4
  PS Constant6/RConn1 -- B13/RConn4
  PS Constant5/RConn1 -- B13/RConn3
  PS Constant7/RConn1 -- B12/RConn3
  PS Constant8/RConn1 -- B12/RConn4
  PS Constant9/RConn1 -- B11/RConn3
  PS Constant12/RConn1 -- B11/RConn4
